simulink model "WaterRunner_nocpg"  (Simulink 8.1)
settings: Solver=ode23s  StartTime=0.0  StopTime=10  RelTol=1e-3
values from neighbouring files (symbols this model uses):
  dTorqueAmp = 0    [simParam.m]    (also in simParam2.m)
  dTorqueFreq = (2*pi)/2    (= 3.14159265359)    [simParam.m]    (also in simParam2.m)
  freq = findSSinput(y,b_water,k_water,A,Fratio,mass*g/4,w0)    [simParam.m]    (also in simParam2.m = 75)
  tail_density = CF_density    (= 1790)    [simParam.m]    (also in simParam2.m)
  tail_length = 0.1    [simParam.m]    (also in simParam2.m)
undefined symbols (not defined in the file or in its folder): X, Y, Z
undefined symbols (not defined in the file): phi0, tail_pad_radius, theta0, water_level, y0
libraries: sm_lib x35, nesl_utility x35, WaterRunner_lib_2 x11, simulink x2
(part 1 of 3)
settings Model: Creator=nitisht  LastModifiedBy=nitisht  SimulationMode=rapid-accelerator
settings SolverCC: ZeroCrossControl=DisableAll  ZeroCrossAlgorithm=Adaptive
settings OptimizationCC: BlockReduction=off  SimCompilerOptimization=On
settings DebuggingCC: SolverPrmCheckMsg=none  FcnCallInpInsideContextMsg=EnableAllAsWarning
settings HardwareCC: ProdBitPerLong=64  ProdBitPerPointer=64  ProdIntDivRoundTo=Zero  ProdEndianess=LittleEndian  ProdWordSize=64  ProdHWDeviceType=Intel->x86-64
settings RTWCC: RTWCompilerOptimization=On
settings GRTTargetCC: CombineOutputUpdateFcns=on  GRTInterface=off
settings ConfigurationSet: Description=SimMechanics 2G
settings ExplorerConfigSet: InternalSimMechanicsExplorerSettings="<ExplorerConfiguration><canonicalview>default</canonicalview><TilePanel><TileInfo><Tiles Columns=\"1\" Count=\"1\" Rows=\"1\"><Column Left=\"2\" Weight=\"1\"/><Column Left=\"1126\"/><Row Top=\"2\" Weight=\"1\"/><Row Top=\"731\"/><Tile Height=\"1\" Width=\"1\" X=\"0\" Y=\"0\"/></Tiles></TileInfo><SceneInfo><SceneViewer><BGColor><R>0.60000002384185791</R><G>0.60000002384185791</G><B>0.60000002384185791</B></BGColor><Camera><Position><X>0.62960776240868022</X><Y>0.44895086159575193</Y><Z>2.4180251146380058</Z></Position><Center><X>0.10015296144366015</X><Y>-0.0072288572057211953</Y><Z>0.36408963188780596</Z></Center><Up><X>-0.10388617680904223</X><Y>0.97626280455059633</Y><Z>-0.19004893769501835</Z></Up><Left>-0.42563784714662656</Left><Right>0.42563784714662656</Right><Bottom>-0.49536256924715738</Bottom><Top>0.49536256924715738</Top></Camera></SceneViewer></SceneInfo></TilePanel></ExplorerConfiguration>"

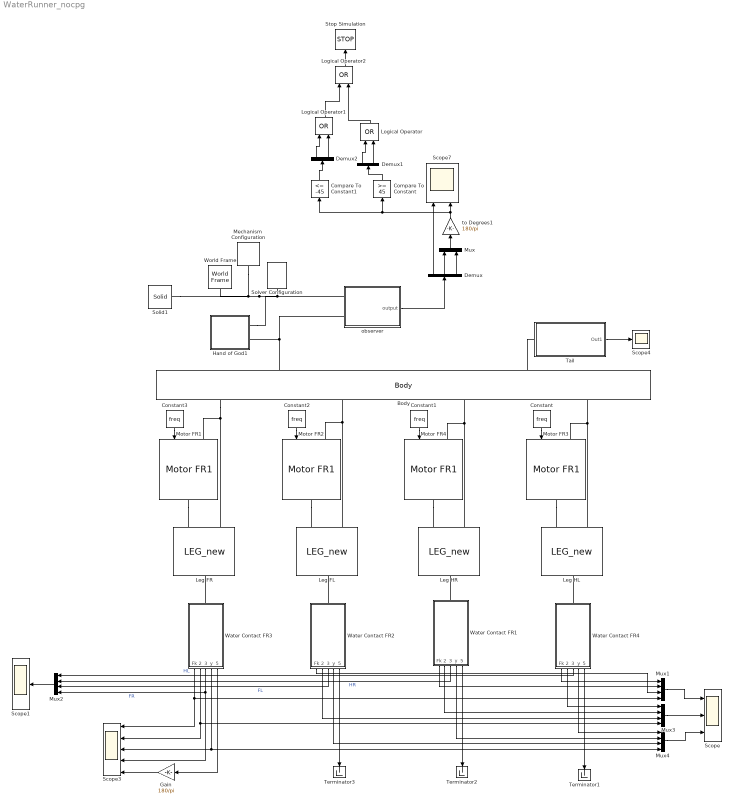
== system WaterRunner_nocpg ==
  Body : WaterRunner_lib_2/Body
  Compare To Constant : simulink/Logic and Bit Operations/Compare To Constant  relop=>=  const=45  OutDataTypeStr=boolean
  Compare To Constant1 : simulink/Logic and Bit Operations/Compare To Constant  relop=<=  const=-45  OutDataTypeStr=boolean
  Constant{,1..3} (4 alike) : Constant  Value=freq
  Demux : Demux  Outputs=3
  Demux1 : Demux  Outputs=2
  Demux2 : Demux  Outputs=2
  Gain : Gain  Gain=180/pi
  Hand of God1 : Subsystem
  Leg FL : WaterRunner_lib_2/LEG_new  p_L1=L1  p_L2=L2  p_L3=L3  p_L4=L4  p_L5=L5  p_CF_density=CF_density  p_bar_w=bar_w  p_bar_h=bar_h  init_pas_ang=0
  Leg FR : WaterRunner_lib_2/LEG_new  p_L1=L1  p_L2=L2  p_L3=L3  p_L4=L4  p_L5=L5  p_CF_density=CF_density  p_bar_w=bar_w  p_bar_h=bar_h  init_pas_ang=0
  Leg HL : WaterRunner_lib_2/LEG_new  p_L1=L1  p_L2=L2  p_L3=L3  p_L4=L4  p_L5=L5  p_CF_density=CF_density  p_bar_w=bar_w  p_bar_h=bar_h  init_pas_ang=0
  Leg HR : WaterRunner_lib_2/LEG_new  p_L1=L1  p_L2=L2  p_L3=L3  p_L4=L4  p_L5=L5  p_CF_density=CF_density  p_bar_w=bar_w  p_bar_h=bar_h  init_pas_ang=0
  Logical Operator : Logic  Operator=OR  AllPortsSameDT=off  OutDataTypeStr=boolean
  Logical Operator1 : Logic  Operator=OR  AllPortsSameDT=off  OutDataTypeStr=boolean
  Logical Operator2 : Logic  Operator=OR  AllPortsSameDT=off  OutDataTypeStr=boolean
  Mechanism  Configuration : sm_lib/Utilities/Mechanism  Configuration  GravityVector=[0 -9.81 0]  GravityUnits=m/s^2  AllowGravitySignal=off  LinearizationDelta=0.001  BlockFunction=simmechanics.library.utilities.mechanism_configuration
  Motor FR1 : WaterRunner_lib_2/Motor FR1  init_ang=180
  Motor FR2 : WaterRunner_lib_2/Motor FR1  init_ang=0
  Motor FR3 : WaterRunner_lib_2/Motor FR1  init_ang=-180
  Motor FR4 : WaterRunner_lib_2/Motor FR1  init_ang=0
  Mux : Mux  Inputs=2
  Mux{1..4} (4 alike) : Mux
  Scope : Scope  NumInputPorts=3
      settings: YMin=0~-2.5~-0.04  YMax=0.325~0.75~0.045
  Scope1 : Scope
      settings: ShowLegends=on  YMin=-2.5  YMax=0.75
  Scope3 : Scope  NumInputPorts=5
      settings: ShowLegends=on  YMin=0~-15~-0.125~-7.5~0  YMax=1.1~2.5~0.1~7.5~130  SaveName=ScopeData4
  Scope4 : Scope
      settings: SaveName=ScopeData2
  Scope7 : Scope  NumInputPorts=2
      settings: TimeRange=10  YMin=-0.015~-45  YMax=0.0175~12.5  SaveName=output
  Solid1 : sm_lib/Body Elements/Solid  InertiaType=PointMass  Mass=0  MassUnits=kg  CenterOfMass=[0 0 0]  CenterOfMassUnits=m  MomentsOfInertia=[1 1 1]  MomentsOfInertiaUnits=kg*m^2  ProductsOfInertia=[0 0 0]  ProductsOfInertiaUnits=kg*m^2  DensityBased=on  Density=1000  DensityUnits=kg/(m^3)  GraphicType=FromGeometry  MarkerShape=Sphere  MarkerSize=10  MarkerSizeUnits=m  GraphicVisPropType=SimpleVisualProperties  GraphicDiffuseColor=[0.4 0.4 1.0]  GraphicSpecularColor=[0.5 0.5 0.5 1.0]  GraphicAmbientColor=[0.15 0.15 0.15 1.0]  GraphicEmissiveColor=[0.0 0.0 0.0 1.0]  GraphicShininess=75  GraphicOpacity=0.5  GeometryShape=Brick  RectangleSize=[1 1]  RectangleSizeUnits=m  BrickDimensions=[20 .001 1]  BrickDimensionUnits=m  CylinderRadius=1  CylinderRadiusUnits=m  CylinderLength=1  CylinderLengthUnits=m  SphereRadius=1  SphereRadiusUnits=m  EllipsoidRadii=[1 1 1]  EllipsoidRadiiUnits=m  ExtrusionCrossSection=[1 1; -1 1; -1 -1; 1 -1]  ExtrusionCrossSectionUnits=m  ExtrusionLength=1  ExtrusionLengthUnits=m  PolygonNumSides=3  PolygonOuterRadius=1  PolygonOuterRadiusUnits=m  ExtGeomFileUnits=m  RevolutionCrossSection=[1 1; 1 -1; 2 -1; 2 1]  RevolutionCrossSectionUnits=m  RevolutionExtent=Full  RevolutionAngle=180  RevolutionAngleUnits=deg  BlockFunction=simmechanics.library.body_elements.solid
  Solver Configuration : nesl_utility/Solver Configuration  PhysicalDomain=network_engine_domain  SubClassName=solver  LeftPortType=input  RightPortType=generic  Accelerate=off  Tones=[]  Harmonics=[]  SimulateNoise=off  Profile=off  UseLocalSampling=off  EnableSwitchedLinearOptims=on  FrequencyDomain=off  UseCCode=off  UseNewInitialization=off  DoDC=off  ResidualTolerance=1e-3  UseLocalSolver=off  LocalSolverChoice=NE_BACKWARD_EULER_ADVANCER  LocalSolverSampleTime=.001  DoFixedCost=off  MaxNonlinIter=3  MaxModeIter=2  LinearAlgebra=Sparse  DelaysMemoryBudget=1024
  Stop Simulation : Stop
  Tail : Subsystem
  Terminator1 : Terminator
  Terminator2 : Terminator
  Terminator3 : Terminator
  Water Contact FR1 : Subsystem  AncestorBlock=WaterRunner_lib_2/Water Contact FR
  Water Contact FR2 : Subsystem  AncestorBlock=WaterRunner_lib_2/Water Contact FR
  Water Contact FR3 : Subsystem  AncestorBlock=WaterRunner_lib_2/Water Contact FR
  Water Contact FR4 : Subsystem  AncestorBlock=WaterRunner_lib_2/Water Contact FR
  World Frame : sm_lib/Frames and  Transforms/World Frame  BlockFunction=simmechanics.library.frames_transforms.world_frame
  observer : Subsystem
  to Degrees1 : Gain  Gain=180/pi
  wires:
  Mux2/1 -> Scope1/1
  Water Contact FR4/3(Vy) -> Mux2/1  "HL"
  Water Contact FR1/3(Vy) -> Mux2/2  "HR"
  Water Contact FR2/3(Vy) -> Mux2/3  "FL"
  Water Contact FR3/3(Vy) -> Scope3/4, Mux2/4  "FR"
  Constant3/1 -> Motor FR1/1
  Constant2/1 -> Motor FR2/1
  Constant1/1 -> Motor FR4/1
  Constant/1 -> Motor FR3/1
  Mux1/1 -> Scope/1
  Mux3/1 -> Scope/2
  Water Contact FR4/1(Fk) -> Mux1/1
  Water Contact FR1/1(Fk) -> Mux1/2
  Water Contact FR2/1(Fk) -> Mux1/3
  Water Contact FR3/1(Fk) -> Mux1/4, Scope3/1
  Water Contact FR4/2(Fb) -> Mux3/1
  Water Contact FR1/2(Fb) -> Mux3/2
  Water Contact FR2/2(Fb) -> Mux3/3
  Water Contact FR3/2(Fb) -> Mux3/4, Scope3/2
  Mux4/1 -> Scope/3
  Water Contact FR4/4(y) -> Mux4/1
  Water Contact FR1/4(y) -> Mux4/2
  Water Contact FR2/4(y) -> Mux4/3
  Water Contact FR3/4(y) -> Mux4/4, Scope3/3
  Water Contact FR3/5(angle) -> Gain/1
  Gain/1 -> Scope3/5
  Tail/1(Out1) -> Scope4/1
  observer/1(output) -> Demux/1
  Demux/2 -> Mux/1
  Demux/3 -> Mux/2
  Mux/1 -> to Degrees1/1
  to Degrees1/1 -> Compare To Constant1/1, Compare To Constant/1, Scope7/2
  Demux/1 -> Scope7/1
  Water Contact FR4/5(angle) -> Terminator1/1
  Water Contact FR1/5(angle) -> Terminator2/1
  Water Contact FR2/5(angle) -> Terminator3/1
  Compare To Constant/1 -> Demux1/1
  Demux1/1 -> Logical Operator/1
  Demux1/2 -> Logical Operator/2
  Compare To Constant1/1 -> Demux2/1
  Demux2/1 -> Logical Operator1/1
  Demux2/2 -> Logical Operator1/2
  Logical Operator1/1 -> Logical Operator2/1
  Logical Operator/1 -> Logical Operator2/2
  Logical Operator2/1 -> Stop Simulation/1
  connections:
  Motor FR1/RConn1 -- Leg FR/LConn1
  Body/LConn1 -- Motor FR1/LConn1 -- Leg FR/LConn2
  Water Contact FR3/LConn1 -- Leg FR/RConn1
  Leg FL/LConn2 -- Motor FR2/LConn1 -- Body/LConn2
  Motor FR2/RConn1 -- Leg FL/LConn1
  Water Contact FR2/LConn1 -- Leg FL/RConn1
  Leg HR/LConn2 -- Motor FR4/LConn1 -- Body/LConn3
  Motor FR4/RConn1 -- Leg HR/LConn1
  Water Contact FR1/LConn1 -- Leg HR/RConn1
  Motor FR3/RConn1 -- Leg HL/LConn1
  Leg HL/LConn2 -- Motor FR3/LConn1 -- Body/LConn4
  Water Contact FR4/LConn1 -- Leg HL/RConn1
  Solver Configuration/RConn1 -- Hand of God1/RConn1 -- Solid1/RConn1 -- World Frame/RConn1 -- Mechanism  Configuration/RConn1 -- observer/LConn1
  Tail/LConn1 -- Body/RConn2
  Body/RConn1 -- Hand of God1/RConn2 -- observer/LConn2

== system WaterRunner_nocpg/Hand of God1 ==
  Product : Product
  Rigid  Transform1 : sm_lib/Frames and  Transforms/Rigid  Transform  TranslationMethod=Cartesian  TranslationLengthUnit=m  TranslationStandardAxis=+Z  TranslationStandardOffset=0  TranslationCartesianOffset=[0 0 0]  TranslationROffset=0  TranslationROffsetUnits=m  TranslationZOffset=0  TranslationZOffsetUnits=m  TranslationThetaOffset=0  TranslationThetaOffsetUnits=deg  RotationMethod=AlignedAxes  RotationAngleUnits=deg  RotationStandardAxis=+Z  RotationAngle=0  RotationArbitraryAxis=[0 0 1]  FollAlignAxisA=+Y  BaseAlignAxisA=+Y  FollAlignAxisB=+Z  BaseAlignAxisB=+X  BlockFunction=simmechanics.library.frames_transforms.rigid_transform
  Rigid  Transform2 : sm_lib/Frames and  Transforms/Rigid  Transform  TranslationMethod=None  TranslationLengthUnit=m  TranslationStandardAxis=+Z  TranslationStandardOffset=0  TranslationCartesianOffset=[0 0 0]  TranslationROffset=0  TranslationROffsetUnits=m  TranslationZOffset=0  TranslationZOffsetUnits=m  TranslationThetaOffset=0  TranslationThetaOffsetUnits=deg  RotationMethod=AlignedAxes  RotationAngleUnits=deg  RotationStandardAxis=+Z  RotationAngle=0  RotationArbitraryAxis=[0 0 1]  FollAlignAxisA=+X  BaseAlignAxisA=+Z  FollAlignAxisB=+Z  BaseAlignAxisB=+Y  BlockFunction=simmechanics.library.frames_transforms.rigid_transform
  Rigid  Transform3 : sm_lib/Frames and  Transforms/Rigid  Transform  TranslationMethod=None  TranslationLengthUnit=m  TranslationStandardAxis=+Z  TranslationStandardOffset=0  TranslationCartesianOffset=[0 0 0]  TranslationROffset=0  TranslationROffsetUnits=m  TranslationZOffset=0  TranslationZOffsetUnits=m  TranslationThetaOffset=0  TranslationThetaOffsetUnits=deg  RotationMethod=AlignedAxes  RotationAngleUnits=deg  RotationStandardAxis=+Z  RotationAngle=0  RotationArbitraryAxis=[0 0 1]  FollAlignAxisA=+Y  BaseAlignAxisA=+Z  FollAlignAxisB=+X  BaseAlignAxisB=+X  BlockFunction=simmechanics.library.frames_transforms.rigid_transform
  Rigid  Transform4 : sm_lib/Frames and  Transforms/Rigid  Transform  TranslationMethod=None  TranslationLengthUnit=m  TranslationStandardAxis=+Z  TranslationStandardOffset=0  TranslationCartesianOffset=[0 0 0]  TranslationROffset=0  TranslationROffsetUnits=m  TranslationZOffset=0  TranslationZOffsetUnits=m  TranslationThetaOffset=0  TranslationThetaOffsetUnits=deg  RotationMethod=AlignedAxes  RotationAngleUnits=deg  RotationStandardAxis=+Z  RotationAngle=0  RotationArbitraryAxis=[0 0 1]  FollAlignAxisA=+Z  BaseAlignAxisA=+X  FollAlignAxisB=+Y  BaseAlignAxisB=+Y  BlockFunction=simmechanics.library.frames_transforms.rigid_transform
  Rigid  Transform5 : sm_lib/Frames and  Transforms/Rigid  Transform  TranslationMethod=None  TranslationLengthUnit=m  TranslationStandardAxis=+Z  TranslationStandardOffset=0  TranslationCartesianOffset=[0 0 0]  TranslationROffset=0  TranslationROffsetUnits=m  TranslationZOffset=0  TranslationZOffsetUnits=m  TranslationThetaOffset=0  TranslationThetaOffsetUnits=deg  RotationMethod=AlignedAxes  RotationAngleUnits=deg  RotationStandardAxis=+Z  RotationAngle=0  RotationArbitraryAxis=[0 0 1]  FollAlignAxisA=+X  BaseAlignAxisA=+Z  FollAlignAxisB=+Z  BaseAlignAxisB=+Y  BlockFunction=simmechanics.library.frames_transforms.rigid_transform
  Rigid  Transform6 : sm_lib/Frames and  Transforms/Rigid  Transform  TranslationMethod=None  TranslationLengthUnit=m  TranslationStandardAxis=+Z  TranslationStandardOffset=0  TranslationCartesianOffset=[0 0 0]  TranslationROffset=0  TranslationROffsetUnits=m  TranslationZOffset=0  TranslationZOffsetUnits=m  TranslationThetaOffset=0  TranslationThetaOffsetUnits=deg  RotationMethod=AlignedAxes  RotationAngleUnits=deg  RotationStandardAxis=+Z  RotationAngle=0  RotationArbitraryAxis=[0 0 1]  FollAlignAxisA=+Z  BaseAlignAxisA=+Y  FollAlignAxisB=+X  BaseAlignAxisB=+X  BlockFunction=simmechanics.library.frames_transforms.rigid_transform
  Scope7 : Scope
      settings: TimeRange=15  YMin=0  YMax=0.001  SaveName=command_omega2
  Simulink-PS Converter : nesl_utility/Simulink-PS Converter  PhysicalDomain=network_engine_domain  SubClassName=ps_input  LeftPortType=input  RightPortType=output  PseudoPeriodic=off  Frequencies=[]  NoiseDistribution=none  NoiseParameters=[]  Unit=1  AffineConversion=off  InputFiltering=off  SimscapeFilterOrder=1  InputFilterTimeConstant=.001  UdotUserProvided=[]
  Sine Wave : Sin  Amplitude=dTorqueAmp  Frequency=dTorqueFreq  SampleTime=0
  Step : Step  Time=3.5  Before=1  After=0  SampleTime=0
  Transport Delay : TransportDelay  DelayTime=2
  forward motion : sm_lib/Joints/Prismatic  Joint  SenseConstraintForceX=off  SenseConstraintForceY=off  SenseConstraintForceZ=off  SenseConstraintTorqueX=off  SenseConstraintTorqueY=off  SenseConstraintTorqueZ=off  ConstraintWrenchDir=FollowerOnBase  ConstraintWrenchFrame=BaseFrame  EquilibriumPosition=0  EquilibriumPositionUnits=m  SpringStiffness=0  SpringStiffnessUnits=N/m  DampingCoefficient=.5  DampingCoefficientUnits=N/(m/s)  ActuationMode=NoActuation  SensePosition=off  SenseVelocity=off  SenseAcceleration=off  SenseTorqueForce=off  PositionTargetValue=0  PositionTargetValueUnits=m  PositionTargetSpecify=on  PositionTargetPriority=High  VelocityTargetValue=2  VelocityTargetValueUnits=m/s  VelocityTargetSpecify=on  VelocityTargetPriority=High  BlockFunction=simmechanics.library.joints.prismatic_joint
  pitch : sm_lib/Joints/Revolute Joint  SenseConstraintForceX=off  SenseConstraintForceY=off  SenseConstraintForceZ=off  SenseConstraintTorqueX=off  SenseConstraintTorqueY=off  SenseConstraintTorqueZ=off  ConstraintWrenchDir=FollowerOnBase  ConstraintWrenchFrame=BaseFrame  EquilibriumPosition=0  EquilibriumPositionUnits=deg  SpringStiffness=0  SpringStiffnessUnits=N*m/deg  DampingCoefficient=0  DampingCoefficientUnits=N*m/(deg/s)  ActuationMode=NoActuation  SensePosition=off  SenseVelocity=off  SenseAcceleration=off  SenseTorqueForce=off  PositionTargetValue=phi0  PositionTargetValueUnits=rad  PositionTargetSpecify=on  PositionTargetPriority=High  VelocityTargetValue=0  VelocityTargetValueUnits=rad/s  VelocityTargetSpecify=on  VelocityTargetPriority=High  BlockFunction=simmechanics.library.joints.revolute_joint
  roll : sm_lib/Joints/Revolute Joint  SenseConstraintForceX=off  SenseConstraintForceY=off  SenseConstraintForceZ=off  SenseConstraintTorqueX=off  SenseConstraintTorqueY=off  SenseConstraintTorqueZ=off  ConstraintWrenchDir=FollowerOnBase  ConstraintWrenchFrame=BaseFrame  EquilibriumPosition=0  EquilibriumPositionUnits=deg  SpringStiffness=0  SpringStiffnessUnits=N*m/deg  DampingCoefficient=0  DampingCoefficientUnits=N*m/(deg/s)  ActuationMode=TorqueForceActuation  SensePosition=off  SenseVelocity=off  SenseAcceleration=off  SenseTorqueForce=off  PositionTargetValue=theta0  PositionTargetValueUnits=rad  PositionTargetSpecify=on  PositionTargetPriority=High  VelocityTargetValue=0  VelocityTargetValueUnits=rad/s  VelocityTargetSpecify=on  VelocityTargetPriority=High  BlockFunction=simmechanics.library.joints.revolute_joint
  up down : sm_lib/Joints/Prismatic  Joint  SenseConstraintForceX=off  SenseConstraintForceY=off  SenseConstraintForceZ=off  SenseConstraintTorqueX=off  SenseConstraintTorqueY=off  SenseConstraintTorqueZ=off  ConstraintWrenchDir=FollowerOnBase  ConstraintWrenchFrame=BaseFrame  EquilibriumPosition=0  EquilibriumPositionUnits=m  SpringStiffness=0  SpringStiffnessUnits=N/m  DampingCoefficient=0  DampingCoefficientUnits=N/(m/s)  ActuationMode=NoActuation  SensePosition=off  SenseVelocity=off  SenseAcceleration=off  SenseTorqueForce=off  PositionTargetValue=y0  PositionTargetValueUnits=m  PositionTargetSpecify=on  PositionTargetPriority=High  VelocityTargetValue=0  VelocityTargetValueUnits=m/s  VelocityTargetSpecify=on  VelocityTargetPriority=High  BlockFunction=simmechanics.library.joints.prismatic_joint
  Base : PMIOPort  Port=1  Side=Right
  Follower : PMIOPort  Port=2  Side=Right
  wires:
  Sine Wave/1 -> Transport Delay/1
  Transport Delay/1 -> Product/2
  Product/1 -> Scope7/1, Simulink-PS Converter/1
  Step/1 -> Product/1
  connections:
  Rigid  Transform1/LConn1 -- Base/RConn1
  Simulink-PS Converter/RConn1 -- roll/LConn2
  Rigid  Transform1/RConn1 -- forward motion/LConn1
  Rigid  Transform4/LConn1 -- pitch/RConn1
  roll/LConn1 -- Rigid  Transform4/RConn1
  forward motion/RConn1 -- Rigid  Transform2/LConn1
  pitch/LConn1 -- Rigid  Transform3/RConn1
  up down/RConn1 -- Rigid  Transform3/LConn1
  Rigid  Transform2/RConn1 -- up down/LConn1
  roll/RConn1 -- Rigid  Transform5/LConn1
  Rigid  Transform5/RConn1 -- Follower/RConn1

== system WaterRunner_nocpg/Tail ==
  PassiveLink : sm_lib/Body Elements/Solid  InertiaType=CalculateFromGeometry  Mass=1  MassUnits=kg  CenterOfMass=[0 0 0]  CenterOfMassUnits=m  MomentsOfInertia=[1 1 1]  MomentsOfInertiaUnits=kg*m^2  ProductsOfInertia=[0 0 0]  ProductsOfInertiaUnits=kg*m^2  DensityBased=on  Density=tail_density*0  DensityUnits=kg/(m^3)  GraphicType=FromGeometry  MarkerShape=Sphere  MarkerSize=10  MarkerSizeUnits=m  GraphicVisPropType=SimpleVisualProperties  GraphicDiffuseColor=[0.4 1.0 0.4]  GraphicSpecularColor=[0.5 0.5 0.5 1.0]  GraphicAmbientColor=[0.15 0.15 0.15 1.0]  GraphicEmissiveColor=[0.0 0.0 0.0 1.0]  GraphicShininess=75  GraphicOpacity=1.0  GeometryShape=Brick  RectangleSize=[1 1]  RectangleSizeUnits=m  BrickDimensions=tail_dim  BrickDimensionUnits=m  CylinderRadius=1  CylinderRadiusUnits=m  CylinderLength=1  CylinderLengthUnits=m  SphereRadius=1  SphereRadiusUnits=m  EllipsoidRadii=[1 1 1]  EllipsoidRadiiUnits=m  ExtrusionCrossSection=[1 1; -1 1; -1 -1; 1 -1]  ExtrusionCrossSectionUnits=m  ExtrusionLength=1  ExtrusionLengthUnits=m  PolygonNumSides=3  PolygonOuterRadius=1  PolygonOuterRadiusUnits=m  ExtGeomFileUnits=m  RevolutionCrossSection=[1 1; 1 -1; 2 -1; 2 1]  RevolutionCrossSectionUnits=m  RevolutionExtent=Full  RevolutionAngle=180  RevolutionAngleUnits=deg  BlockFunction=simmechanics.library.body_elements.solid
  Solid : sm_lib/Body Elements/Solid  InertiaType=PointMass  Mass=0  MassUnits=kg  CenterOfMass=[0 0 0]  CenterOfMassUnits=m  MomentsOfInertia=[1 1 1]  MomentsOfInertiaUnits=kg*m^2  ProductsOfInertia=[0 0 0]  ProductsOfInertiaUnits=kg*m^2  DensityBased=on  Density=0  DensityUnits=kg/(m^3)  GraphicType=FromGeometry  MarkerShape=Sphere  MarkerSize=10  MarkerSizeUnits=m  GraphicVisPropType=SimpleVisualProperties  GraphicDiffuseColor=[0.5 0.5 0.5]  GraphicSpecularColor=[0.5 0.5 0.5 1.0]  GraphicAmbientColor=[0.15 0.15 0.15 1.0]  GraphicEmissiveColor=[0.0 0.0 0.0 1.0]  GraphicShininess=75  GraphicOpacity=1.0  GeometryShape=Cylinder  RectangleSize=[1 1]  RectangleSizeUnits=m  BrickDimensions=[1 1 1]  BrickDimensionUnits=m  CylinderRadius=tail_pad_radius  CylinderRadiusUnits=m  CylinderLength=0.001  CylinderLengthUnits=m  SphereRadius=1  SphereRadiusUnits=m  EllipsoidRadii=[1 1 1]  EllipsoidRadiiUnits=m  ExtrusionCrossSection=[1 1; -1 1; -1 -1; 1 -1]  ExtrusionCrossSectionUnits=m  ExtrusionLength=1  ExtrusionLengthUnits=m  PolygonNumSides=3  PolygonOuterRadius=1  PolygonOuterRadiusUnits=m  ExtGeomFileUnits=m  RevolutionCrossSection=[1 1; 1 -1; 2 -1; 2 1]  RevolutionCrossSectionUnits=m  RevolutionExtent=Full  RevolutionAngle=180  RevolutionAngleUnits=deg  BlockFunction=simmechanics.library.body_elements.solid
  Water Contact HR1 : Subsystem
  pad tran : sm_lib/Frames and  Transforms/Rigid  Transform  TranslationMethod=StandardAxis  TranslationLengthUnit=m  TranslationStandardAxis=-Y  TranslationStandardOffset=0.0015  TranslationCartesianOffset=[0 0 0.25]  TranslationROffset=0  TranslationROffsetUnits=m  TranslationZOffset=0  TranslationZOffsetUnits=m  TranslationThetaOffset=0  TranslationThetaOffsetUnits=deg  RotationMethod=AlignedAxes  RotationAngleUnits=deg  RotationStandardAxis=+Z  RotationAngle=0  RotationArbitraryAxis=[0 0 1]  FollAlignAxisA=+X  BaseAlignAxisA=+X  FollAlignAxisB=+Y  BaseAlignAxisB=+Z  BlockFunction=simmechanics.library.frames_transforms.rigid_transform
  tail_tr_1 : sm_lib/Frames and  Transforms/Rigid  Transform  TranslationMethod=None  TranslationLengthUnit=m  TranslationStandardAxis=+Z  TranslationStandardOffset=0  TranslationCartesianOffset=[0 0 0]  TranslationROffset=0  TranslationROffsetUnits=m  TranslationZOffset=0  TranslationZOffsetUnits=m  TranslationThetaOffset=0  TranslationThetaOffsetUnits=deg  RotationMethod=StandardAxis  RotationAngleUnits=deg  RotationStandardAxis=+Z  RotationAngle=tail_angle  RotationArbitraryAxis=[0 0 1]  FollAlignAxisA=+X  BaseAlignAxisA=+Y  FollAlignAxisB=+Y  BaseAlignAxisB=+Z  BlockFunction=simmechanics.library.frames_transforms.rigid_transform
  tail_tr_2 : sm_lib/Frames and  Transforms/Rigid  Transform  TranslationMethod=StandardAxis  TranslationLengthUnit=m  TranslationStandardAxis=-X  TranslationStandardOffset=tail_length/2  TranslationCartesianOffset=[0 0 0]  TranslationROffset=0  TranslationROffsetUnits=m  TranslationZOffset=0  TranslationZOffsetUnits=m  TranslationThetaOffset=0  TranslationThetaOffsetUnits=deg  RotationMethod=None  RotationAngleUnits=deg  RotationStandardAxis=+Z  RotationAngle=0  RotationArbitraryAxis=[0 0 1]  FollAlignAxisA=+X  BaseAlignAxisA=+Y  FollAlignAxisB=+Y  BaseAlignAxisB=+Z  BlockFunction=simmechanics.library.frames_transforms.rigid_transform
  tail_tr_3 : sm_lib/Frames and  Transforms/Rigid  Transform  TranslationMethod=StandardAxis  TranslationLengthUnit=m  TranslationStandardAxis=-X  TranslationStandardOffset=tail_length/2  TranslationCartesianOffset=[0 0 0]  TranslationROffset=0  TranslationROffsetUnits=m  TranslationZOffset=0  TranslationZOffsetUnits=m  TranslationThetaOffset=0  TranslationThetaOffsetUnits=deg  RotationMethod=None  RotationAngleUnits=deg  RotationStandardAxis=+Z  RotationAngle=0  RotationArbitraryAxis=[0 0 1]  FollAlignAxisA=+X  BaseAlignAxisA=+Y  FollAlignAxisB=+Y  BaseAlignAxisB=+Z  BlockFunction=simmechanics.library.frames_transforms.rigid_transform
  Conn1 : PMIOPort  Port=1  Side=Left
  Out1 : Outport
  wires:
  Water Contact HR1/1(Fb) -> Out1/1
  connections:
  tail_tr_2/LConn1 -- tail_tr_1/RConn1
  tail_tr_2/RConn1 -- PassiveLink/RConn1 -- tail_tr_3/LConn1
  tail_tr_3/RConn1 -- Water Contact HR1/LConn1 -- pad tran/LConn1
  tail_tr_1/LConn1 -- Conn1/RConn1
  pad tran/RConn1 -- Solid/RConn1

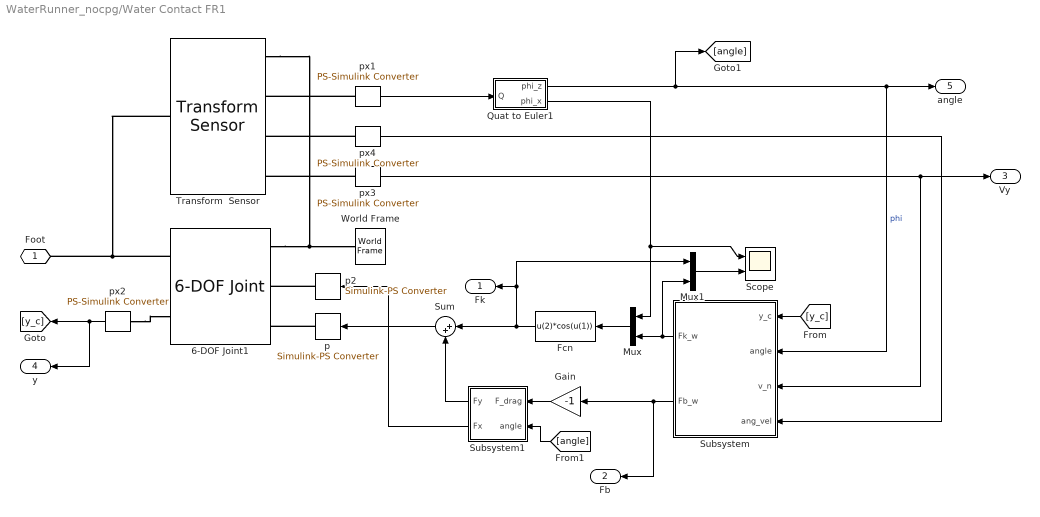
== system WaterRunner_nocpg/Water Contact FR1 ==
  6-DOF Joint1 : sm_lib/Joints/6-DOF Joint  SenseConstraintForceX=off  SenseConstraintForceY=off  SenseConstraintForceZ=off  SenseConstraintTorqueX=off  SenseConstraintTorqueY=off  SenseConstraintTorqueZ=off  ConstraintWrenchDir=FollowerOnBase  ConstraintWrenchFrame=BaseFrame  PxEquilibriumPosition=0  PxEquilibriumPositionUnits=m  PxSpringStiffness=0  PxSpringStiffnessUnits=N/m  PxDampingCoefficient=0  PxDampingCoefficientUnits=N/(m/s)  PxActuationMode=TorqueForceActuation  PxSensePosition=off  PxSenseVelocity=off  PxSenseAcceleration=off  PxSenseTorqueForce=off  PxPositionTargetValue=0  PxPositionTargetValueUnits=m  PxPositionTargetSpecify=off  PxPositionTargetPriority=High  PxVelocityTargetValue=0  PxVelocityTargetValueUnits=m/s  PxVelocityTargetSpecify=off  PxVelocityTargetPriority=High  PyEquilibriumPosition=0  PyEquilibriumPositionUnits=m  PySpringStiffness=0  PySpringStiffnessUnits=N/m  PyDampingCoefficient=0  PyDampingCoefficientUnits=N/(m/s)  PyActuationMode=TorqueForceActuation  PySensePosition=on  PySenseVelocity=off  PySenseAcceleration=off  PySenseTorqueForce=off  PyPositionTargetValue=0  PyPositionTargetValueUnits=m  PyPositionTargetSpecify=off  PyPositionTargetPriority=High  PyVelocityTargetValue=0  PyVelocityTargetValueUnits=m/s  PyVelocityTargetSpecify=off  PyVelocityTargetPriority=High  PzEquilibriumPosition=0  PzEquilibriumPositionUnits=m  PzSpringStiffness=0  PzSpringStiffnessUnits=N/m  PzDampingCoefficient=0  PzDampingCoefficientUnits=N/(m/s)  PzActuationMode=NoActuation  PzSensePosition=off  PzSenseVelocity=off  PzSenseAcceleration=off  PzSenseTorqueForce=off  PzPositionTargetValue=0  PzPositionTargetValueUnits=m  PzPositionTargetSpecify=off  PzPositionTargetPriority=High  PzVelocityTargetValue=0  PzVelocityTargetValueUnits=m/s  PzVelocityTargetSpecify=off  PzVelocityTargetPriority=High  SphDefPosRotationMethod=None  SphDefPosRotationAngleUnits=deg  SphDefPosRotationStandardAxis=+Z  SphDefPosRotationAngle=0  SphDefPosRotationArbitraryAxis=[0 0 1]  SphDefPosFollAlignAxisA=+X  SphDefPosBaseAlignAxisA=+Y  SphDefPosFollAlignAxisB=+Y  SphDefPosBaseAlignAxisB=+Z  SphEqPosRotationMethod=None  SphEqPosRotationAngleUnits=deg  SphEqPosRotationStandardAxis=+Z  SphEqPosRotationAngle=0  SphEqPosRotationArbitraryAxis=[0 0 1]  SphEqPosFollAlignAxisA=+X  SphEqPosBaseAlignAxisA=+Y  SphEqPosFollAlignAxisB=+Y  SphEqPosBaseAlignAxisB=+Z  SphSpringStiffness=0  SphSpringStiffnessUnits=N*m/deg  SphDampingCoefficient=0  SphDampingCoefficientUnits=N*m/(deg/s)  SphActuateTorqueX=off  SphActuateTorqueY=off  SphActuateTorqueZ=off  SphActuateTorque=off  SphActuationMode=NoActuation  SphActuationFrame=BaseFrame  SphSensePosition=off  SphSenseVelocityX=off  SphSenseVelocityY=off  SphSenseVelocityZ=off  SphSenseVelocity=off  SphSenseAccelerationX=off  SphSenseAccelerationY=off  SphSenseAccelerationZ=off  SphSenseAcceleration=off  SphSenseTorqueX=off  SphSenseTorqueY=off  SphSenseTorqueZ=off  SphSenseTorqueForce=off  SphSensingFrame=BaseFrame  SphPositionTargetRotationMethod=None  SphPositionTargetRotationAngleUnits=deg  SphPositionTargetRotationStandardAxis=+Z  SphPositionTargetRotationAngle=0  SphPositionTargetRotationArbitraryAxis=[0 0 1]  SphPositionTargetFollAlignAxisA=+X  SphPositionTargetBaseAlignAxisA=+Y  SphPositionTargetFollAlignAxisB=+Y  SphPositionTargetBaseAlignAxisB=+Z  SphPositionTargetSpecify=off  SphPositionTargetPriority=High  SphVelocityTargetValue=[0 0 0]  SphVelocityTargetValueUnits=deg/s  SphVelocityTargetSpecify=off  SphVelocityTargetPriority=High  SphVelocityTargetInFollowerFrame=on  BlockFunction=simmechanics.library.joints.sixdof_joint
  Fcn : Fcn  Expr=u(2)*cos(u(1))
  Gain : Gain  Gain=-1
  Mux : Mux  Inputs=2
  Mux1 : Mux  Inputs=2
  Quat to Euler1 : Subsystem
  Scope : Scope  NumInputPorts=2
      settings: YMin=-0.19~0  YMax=0.04~0.7  SaveName=ScopeData3
  Subsystem : Subsystem
  Subsystem1 : Subsystem
  Sum : Sum  Inputs=|++
  Transform  Sensor : sm_lib/Frames and  Transforms/Transform  Sensor  MeasurementFrame=NonRotatingBase  SenseAngle=off  SenseAxis=off  SenseAngle1=off  SenseAngle2=off  SenseAngle3=off  SenseQ=on  SenseR=off  SenseOmegaX=off  SenseOmegaY=off  SenseOmegaZ=on  SenseOmega1=off  SenseOmega2=off  SenseOmega3=off  SenseQDot=off  SenseRDot=off  SenseAlphaX=off  SenseAlphaY=off  SenseAlphaZ=off  SenseAlpha1=off  SenseAlpha2=off  SenseAlpha3=off  SenseQDDot=off  SenseRDDot=off  SenseX=off  SenseY=off  SenseZ=off  SenseRad=off  SenseAzim=off  SenseDist=off  SenseInc=off  SenseXDot=off  SenseYDot=on  SenseZDot=off  SenseRadDot=off  SenseAzimDot=off  SenseDistDot=off  SenseIncDot=off  SenseXDDot=off  SenseYDDot=off  SenseZDDot=off  SenseRadDDot=off  SenseAzimDDot=off  SenseDistDDot=off  SenseIncDDot=off  BlockFunction=simmechanics.library.frames_transforms.transform_sensor
  World Frame : sm_lib/Frames and  Transforms/World Frame  BlockFunction=simmechanics.library.frames_transforms.world_frame
  p : nesl_utility/Simulink-PS Converter  PhysicalDomain=network_engine_domain  SubClassName=ps_input  LeftPortType=input  RightPortType=output  PseudoPeriodic=off  Frequencies=[]  NoiseDistribution=none  NoiseParameters=[]  Unit=1  AffineConversion=off  InputFiltering=off  SimscapeFilterOrder=1  InputFilterTimeConstant=.001  UdotUserProvided=[]
  p2 : nesl_utility/Simulink-PS Converter  PhysicalDomain=network_engine_domain  SubClassName=ps_input  LeftPortType=input  RightPortType=output  PseudoPeriodic=off  Frequencies=[]  NoiseDistribution=none  NoiseParameters=[]  Unit=1  AffineConversion=off  InputFiltering=off  SimscapeFilterOrder=1  InputFilterTimeConstant=.001  UdotUserProvided=[]
  px{1..4} (4 alike) : nesl_utility/PS-Simulink Converter  PhysicalDomain=network_engine_domain  SubClassName=ps_output  LeftPortType=input  RightPortType=output  PseudoPeriodic=off  Frequencies=[]  Unit=1  AffineConversion=off
  Foot : PMIOPort  Port=1  Side=Left
  Fk : Outport
  Fb : Outport  Port=2
  Vy : Outport  Port=3
  y : Outport  Port=4
  angle : Outport  Port=5
  wires:
  Subsystem/2(Fb_w) -> Gain/1, Fb/1
  px3/1 -> Vy/1, Subsystem/3(v_n)
  Quat to Euler1/1(phi_z) -> [angle], Subsystem/2(angle), angle/1  "phi"
  px1/1 -> Quat to Euler1/1(Q)
  px4/1 -> Subsystem/4(ang_vel)
  px2/1 -> [y_c], y/1
  [y_c] -> Subsystem/1(y_c)
  [angle] -> Subsystem1/2(angle)
  Sum/1 -> p/1
  Subsystem1/1(Fy) -> Sum/2
  Gain/1 -> Subsystem1/1(F_drag)
  Subsystem1/2(Fx) -> p2/1
  Subsystem/1(Fk_w) -> Mux1/2, Mux/2
  Mux/1 -> Fcn/1
  Fcn/1 -> Mux1/1, Fk/1, Sum/1
  Quat to Euler1/2(phi_x) -> Mux/1, Scope/1
  Mux1/1 -> Scope/2
  connections:
  Transform  Sensor/RConn1 -- World Frame/RConn1 -- 6-DOF Joint1/LConn1
  Transform  Sensor/LConn1 -- Foot/RConn1 -- 6-DOF Joint1/RConn1
  px2/LConn1 -- 6-DOF Joint1/RConn2
  p/RConn1 -- 6-DOF Joint1/LConn3
  px1/LConn1 -- Transform  Sensor/RConn2
  p2/RConn1 -- 6-DOF Joint1/LConn2
  px3/LConn1 -- Transform  Sensor/RConn4
  px4/LConn1 -- Transform  Sensor/RConn3

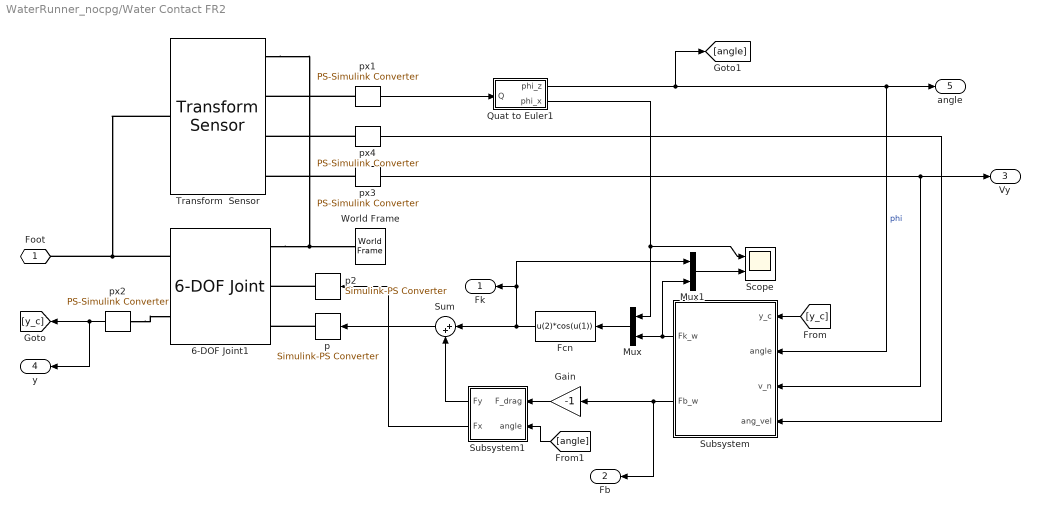
== system WaterRunner_nocpg/Water Contact FR2 ==
  6-DOF Joint1 : sm_lib/Joints/6-DOF Joint  SenseConstraintForceX=off  SenseConstraintForceY=off  SenseConstraintForceZ=off  SenseConstraintTorqueX=off  SenseConstraintTorqueY=off  SenseConstraintTorqueZ=off  ConstraintWrenchDir=FollowerOnBase  ConstraintWrenchFrame=BaseFrame  PxEquilibriumPosition=0  PxEquilibriumPositionUnits=m  PxSpringStiffness=0  PxSpringStiffnessUnits=N/m  PxDampingCoefficient=0  PxDampingCoefficientUnits=N/(m/s)  PxActuationMode=TorqueForceActuation  PxSensePosition=off  PxSenseVelocity=off  PxSenseAcceleration=off  PxSenseTorqueForce=off  PxPositionTargetValue=0  PxPositionTargetValueUnits=m  PxPositionTargetSpecify=off  PxPositionTargetPriority=High  PxVelocityTargetValue=0  PxVelocityTargetValueUnits=m/s  PxVelocityTargetSpecify=off  PxVelocityTargetPriority=High  PyEquilibriumPosition=0  PyEquilibriumPositionUnits=m  PySpringStiffness=0  PySpringStiffnessUnits=N/m  PyDampingCoefficient=0  PyDampingCoefficientUnits=N/(m/s)  PyActuationMode=TorqueForceActuation  PySensePosition=on  PySenseVelocity=off  PySenseAcceleration=off  PySenseTorqueForce=off  PyPositionTargetValue=0  PyPositionTargetValueUnits=m  PyPositionTargetSpecify=off  PyPositionTargetPriority=High  PyVelocityTargetValue=0  PyVelocityTargetValueUnits=m/s  PyVelocityTargetSpecify=off  PyVelocityTargetPriority=High  PzEquilibriumPosition=0  PzEquilibriumPositionUnits=m  PzSpringStiffness=0  PzSpringStiffnessUnits=N/m  PzDampingCoefficient=0  PzDampingCoefficientUnits=N/(m/s)  PzActuationMode=NoActuation  PzSensePosition=off  PzSenseVelocity=off  PzSenseAcceleration=off  PzSenseTorqueForce=off  PzPositionTargetValue=0  PzPositionTargetValueUnits=m  PzPositionTargetSpecify=off  PzPositionTargetPriority=High  PzVelocityTargetValue=0  PzVelocityTargetValueUnits=m/s  PzVelocityTargetSpecify=off  PzVelocityTargetPriority=High  SphDefPosRotationMethod=None  SphDefPosRotationAngleUnits=deg  SphDefPosRotationStandardAxis=+Z  SphDefPosRotationAngle=0  SphDefPosRotationArbitraryAxis=[0 0 1]  SphDefPosFollAlignAxisA=+X  SphDefPosBaseAlignAxisA=+Y  SphDefPosFollAlignAxisB=+Y  SphDefPosBaseAlignAxisB=+Z  SphEqPosRotationMethod=None  SphEqPosRotationAngleUnits=deg  SphEqPosRotationStandardAxis=+Z  SphEqPosRotationAngle=0  SphEqPosRotationArbitraryAxis=[0 0 1]  SphEqPosFollAlignAxisA=+X  SphEqPosBaseAlignAxisA=+Y  SphEqPosFollAlignAxisB=+Y  SphEqPosBaseAlignAxisB=+Z  SphSpringStiffness=0  SphSpringStiffnessUnits=N*m/deg  SphDampingCoefficient=0  SphDampingCoefficientUnits=N*m/(deg/s)  SphActuateTorqueX=off  SphActuateTorqueY=off  SphActuateTorqueZ=off  SphActuateTorque=off  SphActuationMode=NoActuation  SphActuationFrame=BaseFrame  SphSensePosition=off  SphSenseVelocityX=off  SphSenseVelocityY=off  SphSenseVelocityZ=off  SphSenseVelocity=off  SphSenseAccelerationX=off  SphSenseAccelerationY=off  SphSenseAccelerationZ=off  SphSenseAcceleration=off  SphSenseTorqueX=off  SphSenseTorqueY=off  SphSenseTorqueZ=off  SphSenseTorqueForce=off  SphSensingFrame=BaseFrame  SphPositionTargetRotationMethod=None  SphPositionTargetRotationAngleUnits=deg  SphPositionTargetRotationStandardAxis=+Z  SphPositionTargetRotationAngle=0  SphPositionTargetRotationArbitraryAxis=[0 0 1]  SphPositionTargetFollAlignAxisA=+X  SphPositionTargetBaseAlignAxisA=+Y  SphPositionTargetFollAlignAxisB=+Y  SphPositionTargetBaseAlignAxisB=+Z  SphPositionTargetSpecify=off  SphPositionTargetPriority=High  SphVelocityTargetValue=[0 0 0]  SphVelocityTargetValueUnits=deg/s  SphVelocityTargetSpecify=off  SphVelocityTargetPriority=High  SphVelocityTargetInFollowerFrame=on  BlockFunction=simmechanics.library.joints.sixdof_joint
  Fcn : Fcn  Expr=u(2)*cos(u(1))
  Gain : Gain  Gain=-1
  Mux : Mux  Inputs=2
  Mux1 : Mux  Inputs=2
  Quat to Euler1 : Subsystem
  Scope : Scope  NumInputPorts=2
      settings: YMin=-0.19~0  YMax=0.04~0.7  SaveName=ScopeData3
  Subsystem : Subsystem
  Subsystem1 : Subsystem
  Sum : Sum  Inputs=|++
  Transform  Sensor : sm_lib/Frames and  Transforms/Transform  Sensor  MeasurementFrame=NonRotatingBase  SenseAngle=off  SenseAxis=off  SenseAngle1=off  SenseAngle2=off  SenseAngle3=off  SenseQ=on  SenseR=off  SenseOmegaX=off  SenseOmegaY=off  SenseOmegaZ=on  SenseOmega1=off  SenseOmega2=off  SenseOmega3=off  SenseQDot=off  SenseRDot=off  SenseAlphaX=off  SenseAlphaY=off  SenseAlphaZ=off  SenseAlpha1=off  SenseAlpha2=off  SenseAlpha3=off  SenseQDDot=off  SenseRDDot=off  SenseX=off  SenseY=off  SenseZ=off  SenseRad=off  SenseAzim=off  SenseDist=off  SenseInc=off  SenseXDot=off  SenseYDot=on  SenseZDot=off  SenseRadDot=off  SenseAzimDot=off  SenseDistDot=off  SenseIncDot=off  SenseXDDot=off  SenseYDDot=off  SenseZDDot=off  SenseRadDDot=off  SenseAzimDDot=off  SenseDistDDot=off  SenseIncDDot=off  BlockFunction=simmechanics.library.frames_transforms.transform_sensor
  World Frame : sm_lib/Frames and  Transforms/World Frame  BlockFunction=simmechanics.library.frames_transforms.world_frame
  p : nesl_utility/Simulink-PS Converter  PhysicalDomain=network_engine_domain  SubClassName=ps_input  LeftPortType=input  RightPortType=output  PseudoPeriodic=off  Frequencies=[]  NoiseDistribution=none  NoiseParameters=[]  Unit=1  AffineConversion=off  InputFiltering=off  SimscapeFilterOrder=1  InputFilterTimeConstant=.001  UdotUserProvided=[]
  p2 : nesl_utility/Simulink-PS Converter  PhysicalDomain=network_engine_domain  SubClassName=ps_input  LeftPortType=input  RightPortType=output  PseudoPeriodic=off  Frequencies=[]  NoiseDistribution=none  NoiseParameters=[]  Unit=1  AffineConversion=off  InputFiltering=off  SimscapeFilterOrder=1  InputFilterTimeConstant=.001  UdotUserProvided=[]
  px{1..4} (4 alike) : nesl_utility/PS-Simulink Converter  PhysicalDomain=network_engine_domain  SubClassName=ps_output  LeftPortType=input  RightPortType=output  PseudoPeriodic=off  Frequencies=[]  Unit=1  AffineConversion=off
  Foot : PMIOPort  Port=1  Side=Left
  Fk : Outport
  Fb : Outport  Port=2
  Vy : Outport  Port=3
  y : Outport  Port=4
  angle : Outport  Port=5
  wires:
  Subsystem/2(Fb_w) -> Gain/1, Fb/1
  px3/1 -> Vy/1, Subsystem/3(v_n)
  Quat to Euler1/1(phi_z) -> [angle], Subsystem/2(angle), angle/1  "phi"
  px1/1 -> Quat to Euler1/1(Q)
  px4/1 -> Subsystem/4(ang_vel)
  px2/1 -> [y_c], y/1
  [y_c] -> Subsystem/1(y_c)
  [angle] -> Subsystem1/2(angle)
  Sum/1 -> p/1
  Subsystem1/1(Fy) -> Sum/2
  Gain/1 -> Subsystem1/1(F_drag)
  Subsystem1/2(Fx) -> p2/1
  Subsystem/1(Fk_w) -> Mux1/2, Mux/2
  Mux/1 -> Fcn/1
  Fcn/1 -> Mux1/1, Fk/1, Sum/1
  Quat to Euler1/2(phi_x) -> Mux/1, Scope/1
  Mux1/1 -> Scope/2
  connections:
  Transform  Sensor/RConn1 -- World Frame/RConn1 -- 6-DOF Joint1/LConn1
  Transform  Sensor/LConn1 -- Foot/RConn1 -- 6-DOF Joint1/RConn1
  px2/LConn1 -- 6-DOF Joint1/RConn2
  p/RConn1 -- 6-DOF Joint1/LConn3
  px1/LConn1 -- Transform  Sensor/RConn2
  p2/RConn1 -- 6-DOF Joint1/LConn2
  px3/LConn1 -- Transform  Sensor/RConn4
  px4/LConn1 -- Transform  Sensor/RConn3

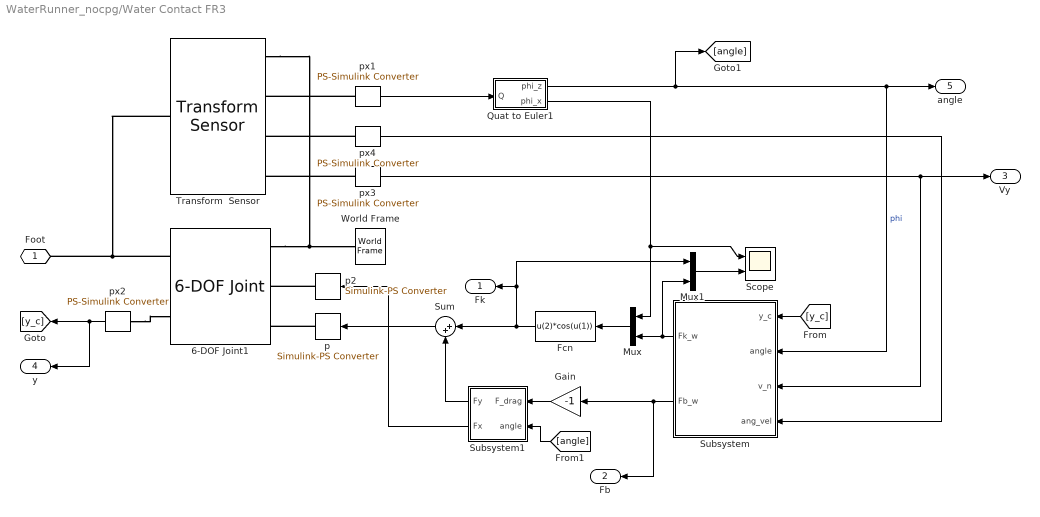
== system WaterRunner_nocpg/Water Contact FR3 ==
  6-DOF Joint1 : sm_lib/Joints/6-DOF Joint  SenseConstraintForceX=off  SenseConstraintForceY=off  SenseConstraintForceZ=off  SenseConstraintTorqueX=off  SenseConstraintTorqueY=off  SenseConstraintTorqueZ=off  ConstraintWrenchDir=FollowerOnBase  ConstraintWrenchFrame=BaseFrame  PxEquilibriumPosition=0  PxEquilibriumPositionUnits=m  PxSpringStiffness=0  PxSpringStiffnessUnits=N/m  PxDampingCoefficient=0  PxDampingCoefficientUnits=N/(m/s)  PxActuationMode=TorqueForceActuation  PxSensePosition=off  PxSenseVelocity=off  PxSenseAcceleration=off  PxSenseTorqueForce=off  PxPositionTargetValue=0  PxPositionTargetValueUnits=m  PxPositionTargetSpecify=off  PxPositionTargetPriority=High  PxVelocityTargetValue=0  PxVelocityTargetValueUnits=m/s  PxVelocityTargetSpecify=off  PxVelocityTargetPriority=High  PyEquilibriumPosition=0  PyEquilibriumPositionUnits=m  PySpringStiffness=0  PySpringStiffnessUnits=N/m  PyDampingCoefficient=0  PyDampingCoefficientUnits=N/(m/s)  PyActuationMode=TorqueForceActuation  PySensePosition=on  PySenseVelocity=off  PySenseAcceleration=off  PySenseTorqueForce=off  PyPositionTargetValue=0  PyPositionTargetValueUnits=m  PyPositionTargetSpecify=off  PyPositionTargetPriority=High  PyVelocityTargetValue=0  PyVelocityTargetValueUnits=m/s  PyVelocityTargetSpecify=off  PyVelocityTargetPriority=High  PzEquilibriumPosition=0  PzEquilibriumPositionUnits=m  PzSpringStiffness=0  PzSpringStiffnessUnits=N/m  PzDampingCoefficient=0  PzDampingCoefficientUnits=N/(m/s)  PzActuationMode=NoActuation  PzSensePosition=off  PzSenseVelocity=off  PzSenseAcceleration=off  PzSenseTorqueForce=off  PzPositionTargetValue=0  PzPositionTargetValueUnits=m  PzPositionTargetSpecify=off  PzPositionTargetPriority=High  PzVelocityTargetValue=0  PzVelocityTargetValueUnits=m/s  PzVelocityTargetSpecify=off  PzVelocityTargetPriority=High  SphDefPosRotationMethod=None  SphDefPosRotationAngleUnits=deg  SphDefPosRotationStandardAxis=+Z  SphDefPosRotationAngle=0  SphDefPosRotationArbitraryAxis=[0 0 1]  SphDefPosFollAlignAxisA=+X  SphDefPosBaseAlignAxisA=+Y  SphDefPosFollAlignAxisB=+Y  SphDefPosBaseAlignAxisB=+Z  SphEqPosRotationMethod=None  SphEqPosRotationAngleUnits=deg  SphEqPosRotationStandardAxis=+Z  SphEqPosRotationAngle=0  SphEqPosRotationArbitraryAxis=[0 0 1]  SphEqPosFollAlignAxisA=+X  SphEqPosBaseAlignAxisA=+Y  SphEqPosFollAlignAxisB=+Y  SphEqPosBaseAlignAxisB=+Z  SphSpringStiffness=0  SphSpringStiffnessUnits=N*m/deg  SphDampingCoefficient=0  SphDampingCoefficientUnits=N*m/(deg/s)  SphActuateTorqueX=off  SphActuateTorqueY=off  SphActuateTorqueZ=off  SphActuateTorque=off  SphActuationMode=NoActuation  SphActuationFrame=BaseFrame  SphSensePosition=off  SphSenseVelocityX=off  SphSenseVelocityY=off  SphSenseVelocityZ=off  SphSenseVelocity=off  SphSenseAccelerationX=off  SphSenseAccelerationY=off  SphSenseAccelerationZ=off  SphSenseAcceleration=off  SphSenseTorqueX=off  SphSenseTorqueY=off  SphSenseTorqueZ=off  SphSenseTorqueForce=off  SphSensingFrame=BaseFrame  SphPositionTargetRotationMethod=None  SphPositionTargetRotationAngleUnits=deg  SphPositionTargetRotationStandardAxis=+Z  SphPositionTargetRotationAngle=0  SphPositionTargetRotationArbitraryAxis=[0 0 1]  SphPositionTargetFollAlignAxisA=+X  SphPositionTargetBaseAlignAxisA=+Y  SphPositionTargetFollAlignAxisB=+Y  SphPositionTargetBaseAlignAxisB=+Z  SphPositionTargetSpecify=off  SphPositionTargetPriority=High  SphVelocityTargetValue=[0 0 0]  SphVelocityTargetValueUnits=deg/s  SphVelocityTargetSpecify=off  SphVelocityTargetPriority=High  SphVelocityTargetInFollowerFrame=on  BlockFunction=simmechanics.library.joints.sixdof_joint
  Fcn : Fcn  Expr=u(2)*cos(u(1))
  Gain : Gain  Gain=-1
  Mux : Mux  Inputs=2
  Mux1 : Mux  Inputs=2
  Quat to Euler1 : Subsystem
  Scope : Scope  NumInputPorts=2
      settings: YMin=-0.19~0  YMax=0.04~0.7  SaveName=ScopeData3
  Subsystem : Subsystem
  Subsystem1 : Subsystem
  Sum : Sum  Inputs=|++
  Transform  Sensor : sm_lib/Frames and  Transforms/Transform  Sensor  MeasurementFrame=NonRotatingBase  SenseAngle=off  SenseAxis=off  SenseAngle1=off  SenseAngle2=off  SenseAngle3=off  SenseQ=on  SenseR=off  SenseOmegaX=off  SenseOmegaY=off  SenseOmegaZ=on  SenseOmega1=off  SenseOmega2=off  SenseOmega3=off  SenseQDot=off  SenseRDot=off  SenseAlphaX=off  SenseAlphaY=off  SenseAlphaZ=off  SenseAlpha1=off  SenseAlpha2=off  SenseAlpha3=off  SenseQDDot=off  SenseRDDot=off  SenseX=off  SenseY=off  SenseZ=off  SenseRad=off  SenseAzim=off  SenseDist=off  SenseInc=off  SenseXDot=off  SenseYDot=on  SenseZDot=off  SenseRadDot=off  SenseAzimDot=off  SenseDistDot=off  SenseIncDot=off  SenseXDDot=off  SenseYDDot=off  SenseZDDot=off  SenseRadDDot=off  SenseAzimDDot=off  SenseDistDDot=off  SenseIncDDot=off  BlockFunction=simmechanics.library.frames_transforms.transform_sensor
  World Frame : sm_lib/Frames and  Transforms/World Frame  BlockFunction=simmechanics.library.frames_transforms.world_frame
  p : nesl_utility/Simulink-PS Converter  PhysicalDomain=network_engine_domain  SubClassName=ps_input  LeftPortType=input  RightPortType=output  PseudoPeriodic=off  Frequencies=[]  NoiseDistribution=none  NoiseParameters=[]  Unit=1  AffineConversion=off  InputFiltering=off  SimscapeFilterOrder=1  InputFilterTimeConstant=.001  UdotUserProvided=[]
  p2 : nesl_utility/Simulink-PS Converter  PhysicalDomain=network_engine_domain  SubClassName=ps_input  LeftPortType=input  RightPortType=output  PseudoPeriodic=off  Frequencies=[]  NoiseDistribution=none  NoiseParameters=[]  Unit=1  AffineConversion=off  InputFiltering=off  SimscapeFilterOrder=1  InputFilterTimeConstant=.001  UdotUserProvided=[]
  px{1..4} (4 alike) : nesl_utility/PS-Simulink Converter  PhysicalDomain=network_engine_domain  SubClassName=ps_output  LeftPortType=input  RightPortType=output  PseudoPeriodic=off  Frequencies=[]  Unit=1  AffineConversion=off
  Foot : PMIOPort  Port=1  Side=Left
  Fk : Outport
  Fb : Outport  Port=2
  Vy : Outport  Port=3
  y : Outport  Port=4
  angle : Outport  Port=5
  wires:
  Subsystem/2(Fb_w) -> Gain/1, Fb/1
  px3/1 -> Vy/1, Subsystem/3(v_n)
  Quat to Euler1/1(phi_z) -> [angle], Subsystem/2(angle), angle/1  "phi"
  px1/1 -> Quat to Euler1/1(Q)
  px4/1 -> Subsystem/4(ang_vel)
  px2/1 -> [y_c], y/1
  [y_c] -> Subsystem/1(y_c)
  [angle] -> Subsystem1/2(angle)
  Sum/1 -> p/1
  Subsystem1/1(Fy) -> Sum/2
  Gain/1 -> Subsystem1/1(F_drag)
  Subsystem1/2(Fx) -> p2/1
  Subsystem/1(Fk_w) -> Mux1/2, Mux/2
  Mux/1 -> Fcn/1
  Fcn/1 -> Mux1/1, Fk/1, Sum/1
  Quat to Euler1/2(phi_x) -> Mux/1, Scope/1
  Mux1/1 -> Scope/2
  connections:
  Transform  Sensor/RConn1 -- World Frame/RConn1 -- 6-DOF Joint1/LConn1
  Transform  Sensor/LConn1 -- Foot/RConn1 -- 6-DOF Joint1/RConn1
  px2/LConn1 -- 6-DOF Joint1/RConn2
  p/RConn1 -- 6-DOF Joint1/LConn3
  px1/LConn1 -- Transform  Sensor/RConn2
  p2/RConn1 -- 6-DOF Joint1/LConn2
  px3/LConn1 -- Transform  Sensor/RConn4
  px4/LConn1 -- Transform  Sensor/RConn3
